simulink model "Lab2_Comparison"  (R2016a)
settings: Solver=VariableStepAuto  StartTime=0.0  StopTime=10.0  RelTol=1e-3
settings Model: Creator=jordan  LastModifiedBy=jordan

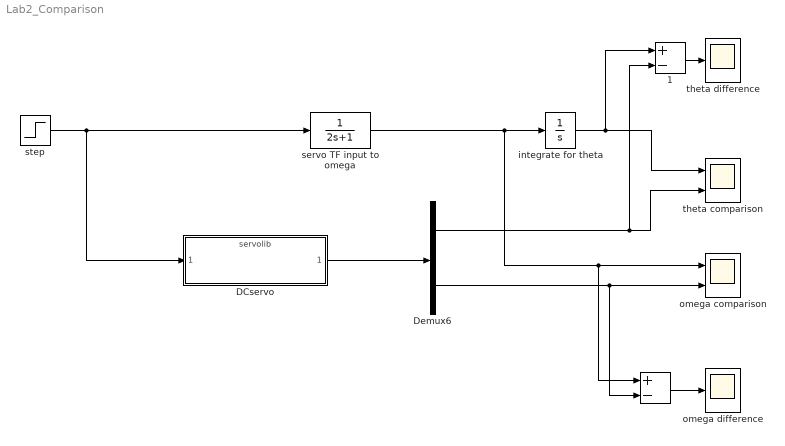
== system Lab2_Comparison ==
  " " : Sum  Inputs=+-
  " 1" : Sum  Inputs=+-
  DCservo : ModelReference  ModelNameDialog=servolib.slx  SimulationMode=Normal  ModelReferenceVersion=1.71
  Demux6 : Demux  Outputs=2
  integrate for theta : TransferFcn  Denominator=[1 0]
  omega comparison : Scope  NumInputPorts=2
  omega difference : Scope
  servo TF input to omega : TransferFcn  Denominator=[2 1]
  step : Step  SampleTime=0
  theta comparison : Scope  NumInputPorts=2
  theta difference : Scope
  wires:
  step/1 -> DCservo/1, servo TF input to omega/1
  Demux6/2 -> " "/2, omega comparison/2
  servo TF input to omega/1 -> integrate for theta/1, " "/1, omega comparison/1
  " "/1 -> omega difference/1
  DCservo/1 -> Demux6/1
  integrate for theta/1 -> " 1"/1, theta comparison/1
  Demux6/1 -> " 1"/2, theta comparison/2
  " 1"/1 -> theta difference/1
